simulink model "lab10_4"  (R2016a)
settings: Solver=VariableStepAuto  StartTime=0.0  StopTime=10.0  RelTol=1e-3
libraries: dspsrcs4 x2
settings Model: Creator=Student  LastModifiedBy=Student

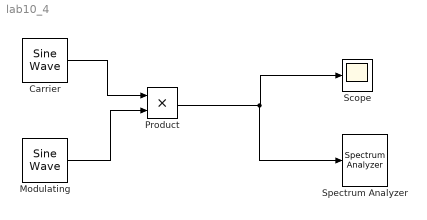
== system lab10_4 ==
  "Carrier " : dspsrcs4/Sine Wave  Amplitude=10  Frequency=50000  Phase=0  SampleMode=Discrete  OutComplex=Real  CompMethod=Trigonometric fcn  TableSize=Speed  SampleTime=1e-6  SamplesPerFrame=1  ResetState=Restart at time zero  OutputFrames=off  dataType=double  wordLen=16  udDataType=sfix(16)  fracBitsMode=Best precision  numFracBits=15  OutDataTypeStr=double  LastOutDataTypeStr=double
  Modulating : dspsrcs4/Sine Wave  Amplitude=0.1  Frequency=2000  Phase=0  SampleMode=Discrete  OutComplex=Real  CompMethod=Trigonometric fcn  TableSize=Speed  SampleTime=1e-6  SamplesPerFrame=1  ResetState=Restart at time zero  OutputFrames=off  dataType=double  wordLen=16  udDataType=sfix(16)  fracBitsMode=Best precision  numFracBits=15  OutDataTypeStr=double  LastOutDataTypeStr=double
  Product : Product
  Scope : Scope
  Spectrum Analyzer : SpectrumAnalyzer
  wires:
  "Carrier "/1 -> Product/1
  Modulating/1 -> Product/2
  Product/1 -> Spectrum Analyzer/1, Scope/1
